simulink model "Commande_c_R2015a"  (R2015a)
settings: Solver=ode45  SolverMode=SingleTasking  StartTime=0.0  StopTime=10  RelTol=1e-3
settings Model: CovMetricSettings=dwe  CovHtmlReporting=off  covSaveCumulativeToWorkspaceVar=off  CovSaveSingleToWorkspaceVar=off  CovExternalEMLEnable=on  Creator=USER  LastModifiedBy=USER
settings DataIOCC: LimitDataPoints=off  SaveFormat=Dataset
settings DebuggingCC: SFUnexpectedBacktrackingDiag=error  SFNoUnconditionalDefaultTransitionDiag=error
settings HardwareCC: ProdBitPerPointer=64  ProdLargestAtomicFloat=Float  ProdIntDivRoundTo=Zero  ProdEndianess=LittleEndian  ProdHWDeviceType=Specified
settings ModelReferenceCC: PropagateSignalLabelsOutOfModel=on
settings SFSimCC: SimUseLocalCustomCode=on
settings RTWCC: RTWUseLocalCustomCode=on
settings GRTTargetCC: TargetLangStandard=C99 (ISO)  GeneratePreprocessorConditionals=Use local settings

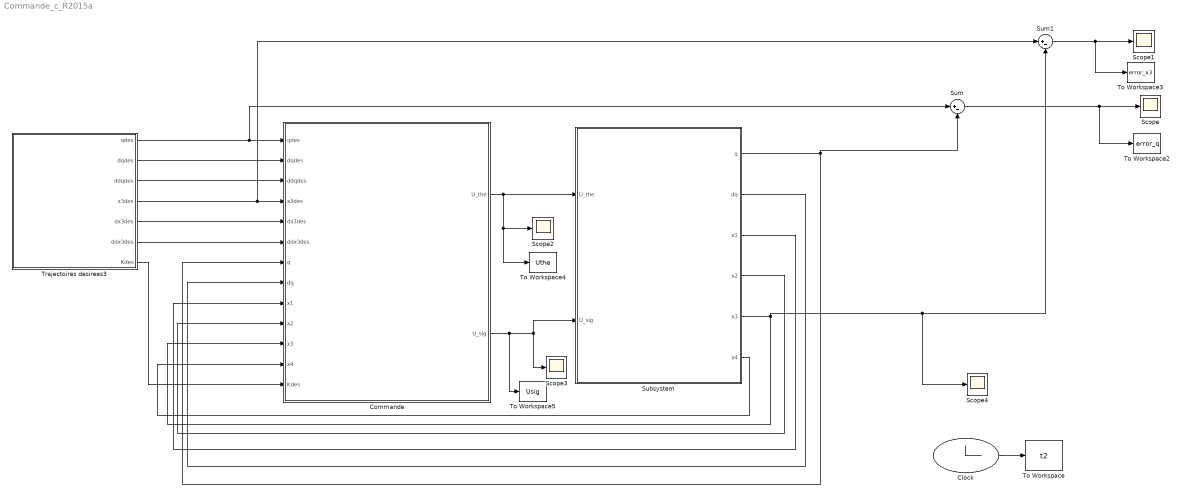
== system Commande_c_R2015a ==
  Clock : Clock
  Commande : Subsystem
  Scope{,1..4} (5 alike) : Scope
      Scope settings: TimeRange=auto  MaxDataPoints=5000  SaveToWorkspace=off  SaveName=ScopeData  YMin=-0.00029  YMax=0.00215  SampleTime=-1
      Scope1 settings: TimeRange=auto  MaxDataPoints=5000  SaveToWorkspace=off  YMin=-0.00715  YMax=0.09813  SampleTime=-1
      Scope2 settings: TimeRange=auto  MaxDataPoints=5000  SaveToWorkspace=off  YMin=-44394.24328  YMax=54683.36507  SampleTime=-1
      Scope3 settings: TimeRange=auto  MaxDataPoints=5000  SaveToWorkspace=off  SaveName=ScopeData2  YMin=-49.02006  YMax=441.18053  SampleTime=-1
      Scope4 settings: TimeRange=auto  MaxDataPoints=5000  SaveToWorkspace=off  YMin=2.829999999996  YMax=2.830000000019  SampleTime=-1
  Subsystem : Subsystem
  Sum : Sum  Inputs=|+-
  Sum1 : Sum  Inputs=|+-
  To Workspace : ToWorkspace  VariableName=t2  SampleTime=-1
  To Workspace2 : ToWorkspace  VariableName=error_q  SampleTime=-1
  To Workspace3 : ToWorkspace  VariableName=error_x3  SampleTime=-1
  To Workspace4 : ToWorkspace  VariableName=Uthe  SampleTime=-1
  To Workspace5 : ToWorkspace  VariableName=Usig  SampleTime=-1
  Trajectoires desirees3 : Subsystem
  wires:
  Trajectoires desirees3/1(qdes) -> Sum/1, Commande/1(qdes)
  Trajectoires desirees3/2(dqdes) -> Commande/2(dqdes)
  Trajectoires desirees3/3(ddqdes) -> Commande/3(ddqdes)
  Trajectoires desirees3/4(x3des) -> Sum1/1, Commande/4(x3des)
  Trajectoires desirees3/5(dx3des) -> Commande/5(dx3des)
  Trajectoires desirees3/6(ddx3des) -> Commande/6(ddx3des)
  Commande/2(U_sig) -> To Workspace5/1, Scope3/1, Subsystem/2(U_sig)
  Subsystem/1(q) -> Commande/7(q), Sum/2
  Subsystem/2(dq) -> Commande/8(dq)
  Subsystem/3(x1) -> Commande/9(x1)
  Subsystem/4(x2) -> Commande/10(x2)
  Subsystem/5(x3) -> Commande/11(x3), Scope4/1, Sum1/2
  Subsystem/6(x4) -> Commande/12(x4)
  Sum/1 -> To Workspace2/1, Scope/1
  Sum1/1 -> To Workspace3/1, Scope1/1
  Trajectoires desirees3/7(Kdes) -> Commande/13(Kdes)
  Commande/1(U_the) -> To Workspace4/1, Scope2/1, Subsystem/1(U_the)
  Clock/1 -> To Workspace/1

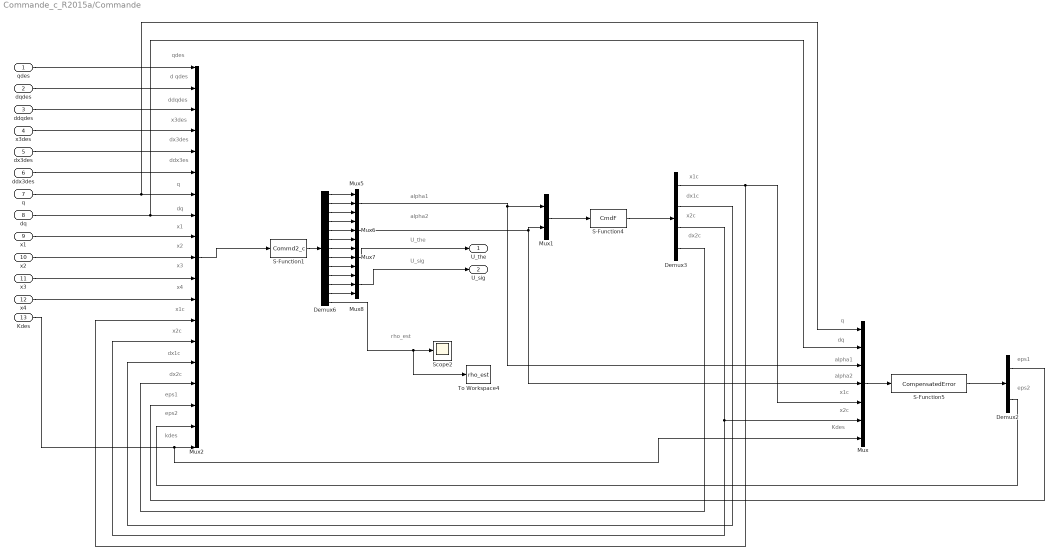
== system Commande_c_R2015a/Commande ==
  note: d qdes
  note: dx2c
  note: dq
  note: ddqdes
  note: x3des
  note: x1c
  note: x1
  note: alpha2
  note: eps2
  note: U_the
  note: eps1
  note: x4
  note: rho_est
  note: alpha1
  note: x1c
  note: U_sig
  note: alpha2
  note: x2c
  note: qdes
  note: x2c
  note: eps1
  note: q
  note: dx1c
  note: x3
  note: Kdes
  note: dq
  note: eps2
  note: ddx3es
  note: x1c
  note: dx3des
  note: dx2c
  note: alpha1
  note: dx1c
  note: q
  note: x2c
  note: x2
  note: kdes
  qdes : Inport
  dqdes : Inport  Port=2
  ddqdes : Inport  Port=3
  x3des : Inport  Port=4
  dx3des : Inport  Port=5
  ddx3des : Inport  Port=6
  q : Inport  Port=7
  dq : Inport  Port=8
  x1 : Inport  Port=9
  x2 : Inport  Port=10
  x3 : Inport  Port=11
  x4 : Inport  Port=12
  Kdes : Inport  Port=13
  Demux2 : Demux  Outputs=2
  Demux3 : Demux
  Demux6 : Demux  Outputs=13
  Mux : Mux  Inputs=7
  Mux1 : Mux  Inputs=2
  Mux2 : Mux  Inputs=19
  Mux{5..8} (4 alike) : Mux  Inputs=3
  S-Function1 : S-Function  FunctionName=Commd2_c  SFunctionDeploymentMode=off  EnableBusSupport=off
  S-Function4 : S-Function  FunctionName=CmdF  SFunctionDeploymentMode=off  EnableBusSupport=off
  S-Function5 : S-Function  FunctionName=CompensatedError  SFunctionDeploymentMode=off  EnableBusSupport=off
  Scope2 : Scope
      settings: TimeRange=auto  MaxDataPoints=5000  SaveToWorkspace=off  YMin=-5.86261  YMax=52.86321  SampleTime=-1
  To Workspace4 : ToWorkspace  VariableName=rho_est  SampleTime=-1
  U_the : Outport
  U_sig : Outport  Port=2
  wires:
  Mux1/1 -> S-Function4/1
  S-Function5/1 -> Demux2/1
  Mux6/1 -> Mux/4, Mux1/2
  S-Function4/1 -> Demux3/1
  Mux2/1 -> S-Function1/1
  Mux5/1 -> Mux1/1, Mux/3
  Mux/1 -> S-Function5/1
  Mux7/1 -> U_the/1
  Mux8/1 -> U_sig/1
  Demux3/1 -> Mux2/13, Mux/5
  Demux3/3 -> Mux2/14, Mux/6
  Demux6/13 -> To Workspace4/1, Scope2/1
  Demux6/3 -> Mux5/3
  Demux6/2 -> Mux5/2
  Demux6/4 -> Mux6/1
  Demux6/5 -> Mux6/2
  Demux6/6 -> Mux6/3
  Demux6/1 -> Mux5/1
  Demux6/9 -> Mux7/3
  S-Function1/1 -> Demux6/1
  Demux6/8 -> Mux7/2
  Demux6/10 -> Mux8/1
  Demux6/11 -> Mux8/2
  Demux6/12 -> Mux8/3
  Demux6/7 -> Mux7/1
  qdes/1 -> Mux2/1
  dqdes/1 -> Mux2/2
  ddqdes/1 -> Mux2/3
  x3des/1 -> Mux2/4
  dx3des/1 -> Mux2/5
  ddx3des/1 -> Mux2/6
  q/1 -> Mux2/7, Mux/1
  dq/1 -> Mux/2, Mux2/8
  x1/1 -> Mux2/9
  x2/1 -> Mux2/10
  x3/1 -> Mux2/11
  x4/1 -> Mux2/12
  Demux3/2 -> Mux2/15
  Demux3/4 -> Mux2/16
  Demux2/1 -> Mux2/17
  Demux2/2 -> Mux2/18
  Kdes/1 -> Mux/7, Mux2/19

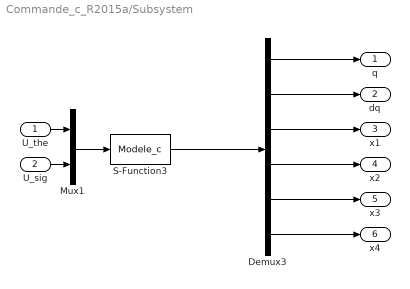
== system Commande_c_R2015a/Subsystem ==
  U_the : Inport
  U_sig : Inport  Port=2
  Demux3 : Demux  Outputs=6
  Mux1 : Mux  Inputs=2
  S-Function3 : S-Function  FunctionName=Modele_c  SFunctionDeploymentMode=off  EnableBusSupport=off
  q : Outport
  dq : Outport  Port=2
  x1 : Outport  Port=3
  x2 : Outport  Port=4
  x3 : Outport  Port=5
  x4 : Outport  Port=6
  wires:
  Mux1/1 -> S-Function3/1
  U_the/1 -> Mux1/1
  U_sig/1 -> Mux1/2
  S-Function3/1 -> Demux3/1
  Demux3/1 -> q/1
  Demux3/2 -> dq/1
  Demux3/3 -> x1/1
  Demux3/4 -> x2/1
  Demux3/5 -> x3/1
  Demux3/6 -> x4/1

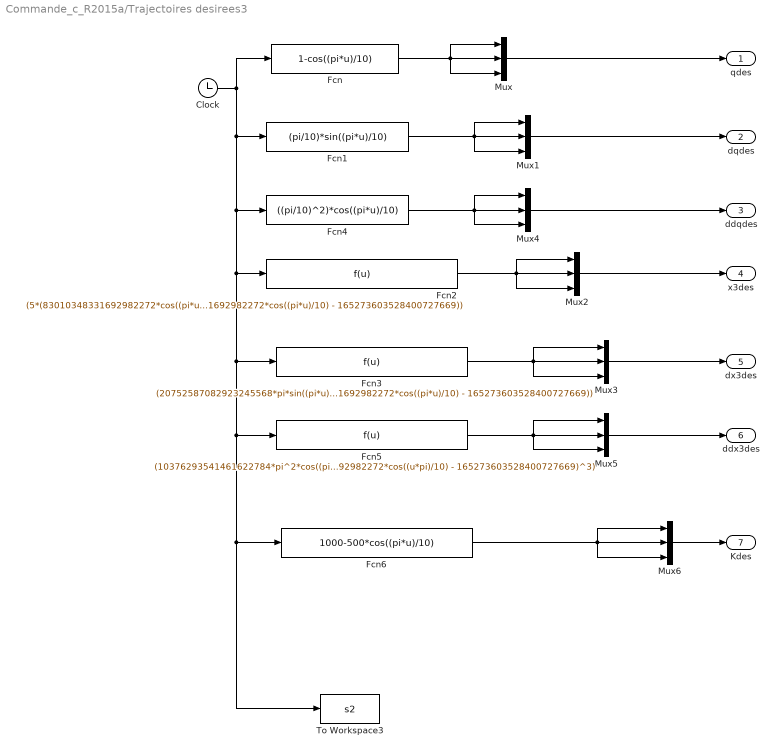
== system Commande_c_R2015a/Trajectoires desirees3 ==
  Clock : Clock
  Fcn : Fcn  Expr=1-cos((pi*u)/10)
  Fcn1 : Fcn  Expr=(pi/10)*sin((pi*u)/10)
  Fcn2 : Fcn  Expr=(5*(83010348331692982272*cos((pi*u)/10) + 149418626997047375*(166020696663385964544/29883725399409475 - (83010348331692982272*cos((pi*u)/10))/29883725399409475)^(1/2) - 166020696663385964544))/(2*(83010348331692982272*cos((pi*u)/10) - 165273603528400727669))
  Fcn3 : Fcn  Expr=(20752587082923245568*pi*sin((pi*u)/10)*(83010348331692982272*cos((pi*u)/10) + 149418626997047375*(166020696663385964544/29883725399409475 - (83010348331692982272*cos((pi*u)/10))/29883725399409475)^(1/2) - 166020696663385964544))/(83010348331692982272*cos((u*pi)/10) - 165273603528400727669)^2 - (5*((41505174165846491136*pi*sin((pi*u)/10))/5 - (20752587082923245568*pi*sin((pi*u)/10))/(- (83010348331692982272*cos((u*pi)/10))/29883725399409475 + 166020696663385964544/29883725399409475)^(1/2)))/(2*(83010348331692982272*cos((pi*u)/10) - 165273603528400727669))
  Fcn4 : Fcn  Expr=((pi/10)^2)*cos((pi*u)/10)
  Fcn5 : Fcn  Expr=(10376293541461622784*pi^2*cos((pi*u)/10)*(83010348331692982272*cos((pi*u)/10) + 149418626997047375*(166020696663385964544/29883725399409475 - (83010348331692982272*cos((pi*u)/10))/29883725399409475)^(1/2) - 166020696663385964544))/(5*(83010348331692982272*cos((u*pi)/10) - 165273603528400727669)^2) - (41505174165846491136*pi*sin((pi*u)/10)*((41505174165846491136*pi*sin((pi*u)/10))/5 - (20752587082923245568*pi*sin((pi*u)/10))/(- (83010348331692982272*cos((u*pi)/10))/29883725399409475 + 166020696663385964544/29883725399409475)^(1/2)))/(83010348331692982272*cos((u*pi)/10) - 165273603528400727669)^2 - (5*((20752587082923245568*pi^2*cos((pi*u)/10))/25 - (10376293541461622784*pi^2*cos((pi*u)/10))/(5*(- (83010348331692982272*cos((u*pi)/10))/29883725399409475 + 166020696663385964544/29883725399409475)^(1/2)) + (430669870634312742820833487530831642624*pi^2*sin((pi*u)/10)^2)/(149418626997047375*(- (83010348331692982272*cos((u*pi)/10))/29883725399409475 + 166020696663385964544/29883725399409475)^(3/2))))/(2*(83010348331692982272*cos((pi*u)/10) - 165273603528400727669)) + (1722679482537250971283333950123326570496*pi^2*sin((pi*u)/10)^2*(83010348331692982272*cos((pi*u)/10) + 149418626997047375*(166020696663385964544/29883725399409475 - (83010348331692982272*cos((pi*u)/10))/29883725399409475)^(1/2) - 166020696663385964544))/(5*(83010348331692982272*cos((u*pi)/10) - 165273603528400727669)^3)
  Fcn6 : Fcn  Expr=1000-500*cos((pi*u)/10)
  Mux{,1..6} (7 alike) : Mux  Inputs=3
  To Workspace3 : ToWorkspace  VariableName=s2  SampleTime=-1
  qdes : Outport
  dqdes : Outport  Port=2
  ddqdes : Outport  Port=3
  x3des : Outport  Port=4
  dx3des : Outport  Port=5
  ddx3des : Outport  Port=6
  Kdes : Outport  Port=7
  wires:
  Fcn/1 -> Mux/3, Mux/2, Mux/1
  Fcn1/1 -> Mux1/3, Mux1/1, Mux1/2
  Fcn2/1 -> Mux2/3, Mux2/2, Mux2/1
  Fcn3/1 -> Mux3/3, Mux3/2, Mux3/1
  Mux3/1 -> dx3des/1
  Mux2/1 -> x3des/1
  Mux1/1 -> dqdes/1
  Mux/1 -> qdes/1
  Fcn4/1 -> Mux4/3, Mux4/1, Mux4/2
  Mux4/1 -> ddqdes/1
  Mux5/1 -> ddx3des/1
  Fcn5/1 -> Mux5/3, Mux5/2, Mux5/1
  Fcn6/1 -> Mux6/1, Mux6/3, Mux6/2
  Mux6/1 -> Kdes/1
  Clock/1 -> Fcn6/1, To Workspace3/1, Fcn5/1, Fcn3/1, Fcn2/1, Fcn4/1, Fcn1/1, Fcn/1
